simulink model "transformer_rectifier_unit"  (R2014a)
settings: Solver=FixedStepDiscrete  SolverMode=SingleTasking  StartTime=0.0  StopTime=5  FixedStep=Ts  MaxStep=1e-3  RelTol=1e-4  AbsTol=1e-4
PreLoadFcn:
  | Ts = 4e-5;
StartFcn:
  | tic;
StopFcn:
  | toc;
undefined symbols (not defined in the file or in its folder): DiscIntNeverNeededParam, param
libraries: powerlib x32, powerlib_meascontrol x5, simulink x4
settings Model: Creator=abennett  LastModifiedBy=cosorio
settings DataIOCC: SaveOutput=off  SaveTime=off  SignalLoggingName=TRU_Data
settings OptimizationCC: ExpressionDepthLimit=2147483647
settings DebuggingCC: UnderspecifiedInitializationDetection=Classic  FcnCallInpInsideContextMsg=UseLocalSettings  StateNameClashWarn=warning
settings GRTTargetCC: CombineOutputUpdateFcns=off  GRTInterface=on

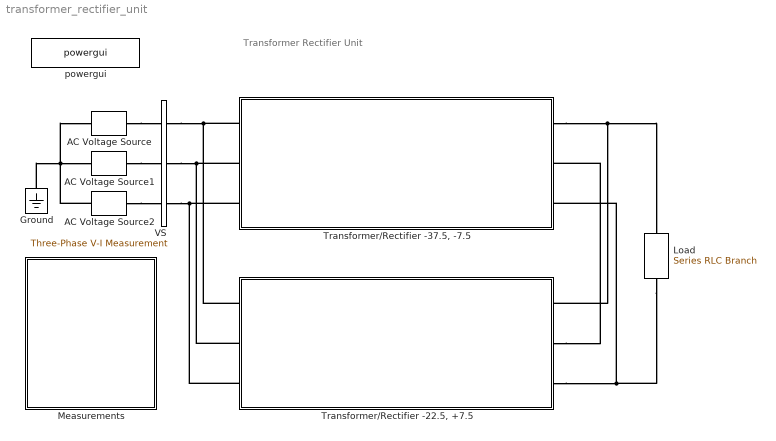
== system transformer_rectifier_unit ==
  note: Transformer Rectifier Unit
  AC Voltage Source : powerlib/Electrical Sources/AC Voltage Source  Amplitude=6600*sqrt(2)/sqrt(3)  Phase=0  Frequency=60  SampleTime=Ts  Measurements=None
  AC Voltage Source1 : powerlib/Electrical Sources/AC Voltage Source  Amplitude=6600*sqrt(2)/sqrt(3)  Phase=-120  Frequency=60  SampleTime=Ts  Measurements=None
  AC Voltage Source2 : powerlib/Electrical Sources/AC Voltage Source  Amplitude=6600*sqrt(2)/sqrt(3)  Phase=120  Frequency=60  SampleTime=Ts  Measurements=None
  Ground : powerlib/Elements/Ground  LConnTagsString=a
  Load : powerlib/Elements/Series RLC Branch  LConnTagsString=__new0  RConnTagsString=__new0  BranchType=R  Resistance=1  Inductance=1e-3  SetiL0=off  InitialCurrent=0  Capacitance=param.conv.C1  Setx0=off  InitialVoltage=0  Measurements=Branch voltage and current
  Measurements : Subsystem
  "Transformer/Rectifier -22.5, +7.5" : Subsystem
  "Transformer/Rectifier -37.5, -7.5" : Subsystem
  VS : powerlib/Measurements/Three-Phase V-I Measurement  VoltageMeasurement=phase-to-phase  SetLabelV=on  LabelV=Vsupply  Vpu=off  VpuLL=off  CurrentMeasurement=yes  SetLabelI=on  LabelI=Isupply  Ipu=off  Pbase=100e6  Vbase=500e3  OutputType=Complex  PhasorSimulation=off  PSBequivalent=0
  powergui : powerlib/powergui  Priority=1  SimulationMode=Discrete  SolverType=Tustin  SampleTime=Ts  frequency=60  SPID=off  DisableSnubberDevices=on  DisableRonSwitches=on  DisableVfSwitches=on  SwTol=0  Interpol=off  DisplayEquations=off  Ts=0  methode=off  frequencyindice=60  Pbase=100e6  ErrMax=1e-4  Iterations=50  UnitsV=kV  UnitsW=MW  FunctionMessages=off  echomessages=off  HookPort=off  EnableUseOfTLC=off  x0status=blocks  RestoreLinks=warning  ResistiveCurrentMeasurement=off  Frange=[0:2:500]  Ylog=off  Xlog=on  ShowGrid=off  save=off  variable=ZData  structure=VISupply  ZoomFFT=off  StartTime=2  cycles=10  DisplayStyle=1  fundamental=60  FreqAxis=on  MaxFrequency=3600  frequencyindicesteady=1  RmsSteady=1  display=off
  connections:
  VS/RConn1 -- "Transformer/Rectifier -22.5, +7.5"/LConn1 -- "Transformer/Rectifier -37.5, -7.5"/LConn1
  VS/RConn2 -- "Transformer/Rectifier -22.5, +7.5"/LConn2 -- "Transformer/Rectifier -37.5, -7.5"/LConn2
  VS/RConn3 -- "Transformer/Rectifier -22.5, +7.5"/LConn3 -- "Transformer/Rectifier -37.5, -7.5"/LConn3
  "Transformer/Rectifier -37.5, -7.5"/RConn1 -- Load/LConn1 -- "Transformer/Rectifier -22.5, +7.5"/RConn1
  Load/RConn1 -- "Transformer/Rectifier -22.5, +7.5"/RConn3 -- "Transformer/Rectifier -37.5, -7.5"/RConn3
  "Transformer/Rectifier -22.5, +7.5"/RConn2 -- "Transformer/Rectifier -37.5, -7.5"/RConn2
  AC Voltage Source2/RConn1 -- VS/LConn3
  AC Voltage Source1/RConn1 -- VS/LConn2
  AC Voltage Source/RConn1 -- VS/LConn1
  AC Voltage Source2/LConn1 -- Ground/LConn1 -- AC Voltage Source1/LConn1 -- AC Voltage Source/LConn1

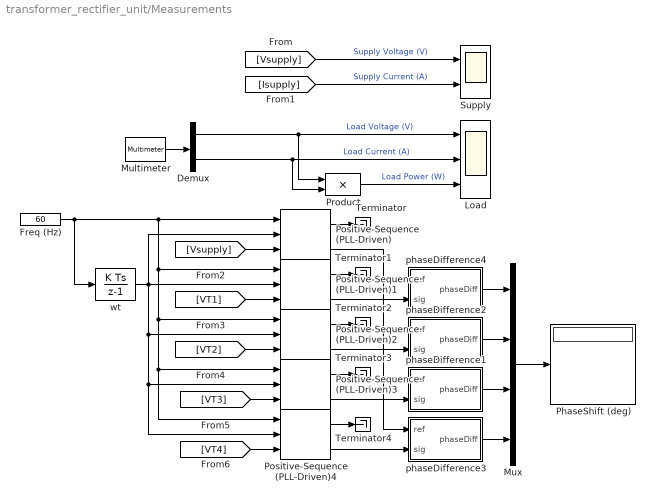
== system transformer_rectifier_unit/Measurements ==
  Demux : Demux  Outputs=2
  Freq (Hz) : Constant  Value=60
  Load : Scope  NumInputPorts=3
      settings: YMin=0~0~0  YMax=3000~3000~5000000  SaveName=VILoad
  Multimeter : powerlib/Measurements/Multimeter  PhasorSimulation=off  OutputType=Complex  sel=[1 2]  L=2  Gain=[1 1]  yselected={'Ub: Load','Ib: Load'};  PSBOutputType=1  PSBequivalent=0  AxesSetting=[0,0.1,-100,100]  Display=0  SavedBlockNames=-11
  Mux : Mux
  PhaseShift (deg) : Display
      settings: Format=bank  Decimation=100
  Positive-Sequence (PLL-Driven){,1..4} (5 alike) : powerlib_meascontrol/Measurements/Positive-Sequence (PLL-Driven)  Finit=60  Fmin=45  InInit=[1, 0]  Ts=Ts
  Product : Product  RndMeth=Zero
  Supply : Scope  NumInputPorts=2
      settings: YMin=-15000~-1000  YMax=15000~1000  SaveName=VISupply
  Terminator{,1..4} (5 alike) : Terminator
  phaseDifference1 : Subsystem
  phaseDifference2 : Subsystem
  phaseDifference3 : Subsystem
  phaseDifference4 : Subsystem
  wt : DiscreteIntegrator  gainval=2*pi  SampleTime=Ts  ICPrevOutput=DiscIntNeverNeededParam  ICPrevScaledInput=DiscIntNeverNeededParam
  wires:
  [Vsupply] -> Supply/1  "Supply Voltage (V)"
  [Isupply] -> Supply/2  "Supply Current (A)"
  Multimeter/1 -> Demux/1
  Demux/1 -> Product/1, Load/1  "Load Voltage (V)"
  Demux/2 -> Product/2, Load/2  "Load Current (A)"
  Product/1 -> Load/3  "Load Power (W)"
  [Vsupply] -> Positive-Sequence (PLL-Driven)/3
  [VT1] -> Positive-Sequence (PLL-Driven)1/3
  [VT2] -> Positive-Sequence (PLL-Driven)2/3
  [VT4] -> Positive-Sequence (PLL-Driven)4/3
  Positive-Sequence (PLL-Driven)/2 -> phaseDifference4/1(ref), phaseDifference2/1(ref), phaseDifference1/1(ref), phaseDifference3/1(ref)
  Positive-Sequence (PLL-Driven)1/2 -> phaseDifference4/2(sig)
  Positive-Sequence (PLL-Driven)2/2 -> phaseDifference2/2(sig)
  Positive-Sequence (PLL-Driven)4/2 -> phaseDifference3/2(sig)
  Positive-Sequence (PLL-Driven)/1 -> Terminator/1
  Positive-Sequence (PLL-Driven)1/1 -> Terminator1/1
  Positive-Sequence (PLL-Driven)2/1 -> Terminator2/1
  Positive-Sequence (PLL-Driven)3/1 -> Terminator3/1
  phaseDifference4/1(phaseDiff) -> Mux/1
  phaseDifference2/1(phaseDiff) -> Mux/2
  phaseDifference1/1(phaseDiff) -> Mux/3
  phaseDifference3/1(phaseDiff) -> Mux/4
  Mux/1 -> PhaseShift (deg)/1
  Positive-Sequence (PLL-Driven)4/1 -> Terminator4/1
  Positive-Sequence (PLL-Driven)3/2 -> phaseDifference1/2(sig)
  [VT3] -> Positive-Sequence (PLL-Driven)3/3
  Freq (Hz)/1 -> Positive-Sequence (PLL-Driven)4/1, Positive-Sequence (PLL-Driven)3/1, Positive-Sequence (PLL-Driven)2/1, Positive-Sequence (PLL-Driven)1/1, Positive-Sequence (PLL-Driven)/1, wt/1
  wt/1 -> Positive-Sequence (PLL-Driven)/2, Positive-Sequence (PLL-Driven)1/2, Positive-Sequence (PLL-Driven)2/2, Positive-Sequence (PLL-Driven)3/2, Positive-Sequence (PLL-Driven)4/2

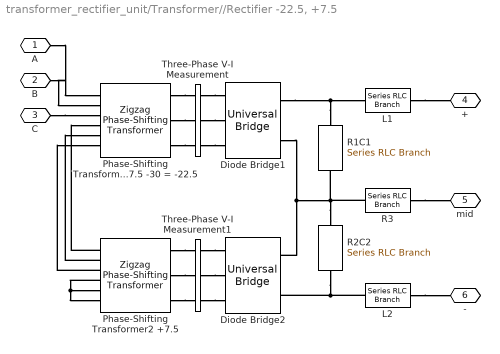
== system transformer_rectifier_unit/Transformer//Rectifier -22.5, +7.5 ==
  Diode Bridge1 : powerlib/Power Electronics/Universal Bridge  Arms=3  SnubberResistance=80  SnubberCapacitance=1e-06  Device=Diodes  Ron=1e-3  Lon=0  ForwardVoltages="[  0  0  ]"  ForwardVoltage=0  GTOparameters=[ 10e-6 , 20e-6 ]  IGBTparameters=[ 1e-6 , 2e-6 ]  Measurements=None  Measurements_2=None  converterType=Rectifier
  Diode Bridge2 : powerlib/Power Electronics/Universal Bridge  Arms=3  SnubberResistance=80  SnubberCapacitance=1e-06  Device=Diodes  Ron=1e-3  Lon=0  ForwardVoltages="[  0  0  ]"  ForwardVoltage=0  GTOparameters=[ 10e-6 , 20e-6 ]  IGBTparameters=[ 1e-6 , 2e-6 ]  Measurements=None  Measurements_2=None  converterType=Rectifier
  L1 : powerlib/Elements/Series RLC Branch  LConnTagsString=__new0  RConnTagsString=__new0  BranchType=L  Resistance=param.conv.R3  Inductance=0.005e-3  SetiL0=off  InitialCurrent=0  Capacitance=param.conv.C1  Setx0=off  InitialVoltage=0  Measurements=None
  L2 : powerlib/Elements/Series RLC Branch  LConnTagsString=__new0  RConnTagsString=__new0  BranchType=L  Resistance=param.conv.R3  Inductance=0.005e-3  SetiL0=off  InitialCurrent=0  Capacitance=param.conv.C1  Setx0=off  InitialVoltage=0  Measurements=None
  Phase-Shifting Transformer1 +7.5 -30 = -22.5 : powerlib/Elements/Zigzag Phase-Shifting Transformer  SecondaryConnection=Delta D1(-30 deg.)  UNITS=pu  NominalPower=[3300e3 60]  PrimaryVoltage=6600  SecondaryVoltage="[1725  7.5]"  Winding1=[ 0.002 0.08 ]  Winding2="[ 0.002  0.08 ]"  Winding3=[ 0.002 0.08 ]  SetSaturation=off  RmLm=[ 500 500 ]  Rm=500  Saturation=[ 0,0 ; 0.0024,1.2 ; 1.0,1.52 ]  SetInitialFlux=off  Measurements=None  InitialFluxes=[0,0,0]  MoreParameters=on  BreakLoop=off  DataType=off
  Phase-Shifting Transformer2 +7.5 : powerlib/Elements/Zigzag Phase-Shifting Transformer  SecondaryConnection=Y  UNITS=pu  NominalPower=[3300e3 60]  PrimaryVoltage=6600  SecondaryVoltage="[1725  7.5]"  Winding1=[ 0.002 0.08 ]  Winding2="[ 0.002  0.08 ]"  Winding3=[ 0.002 0.08 ]  SetSaturation=off  RmLm=[ 500 500 ]  Rm=500  Saturation=[ 0,0 ; 0.0024,1.2 ; 1.0,1.52 ]  SetInitialFlux=off  Measurements=None  InitialFluxes=[0,0,0]  MoreParameters=on  BreakLoop=off  DataType=off
  R1C1 : powerlib/Elements/Series RLC Branch  LConnTagsString=__new0  RConnTagsString=__new0  BranchType=RC  Resistance=2.5  Inductance=1e-3  SetiL0=off  InitialCurrent=0  Capacitance=10e-6  Setx0=off  InitialVoltage=0  Measurements=None
  R2C2 : powerlib/Elements/Series RLC Branch  LConnTagsString=__new0  RConnTagsString=__new0  BranchType=RC  Resistance=2.5  Inductance=1e-3  SetiL0=off  InitialCurrent=0  Capacitance=10e-6  Setx0=off  InitialVoltage=0  Measurements=None
  R3 : powerlib/Elements/Series RLC Branch  LConnTagsString=__new0  RConnTagsString=__new0  BranchType=R  Resistance=10e3  Inductance=1e-3  SetiL0=off  InitialCurrent=0  Capacitance=param.conv.C1  Setx0=off  InitialVoltage=0  Measurements=None
  Three-Phase V-I Measurement : powerlib/Measurements/Three-Phase V-I Measurement  VoltageMeasurement=phase-to-phase  SetLabelV=on  LabelV=VT3  Vpu=off  VpuLL=off  CurrentMeasurement=no  SetLabelI=off  LabelI=Iabc  Ipu=off  Pbase=100e6  Vbase=500e3  OutputType=Complex  PhasorSimulation=off  PSBequivalent=0
  Three-Phase V-I Measurement1 : powerlib/Measurements/Three-Phase V-I Measurement  VoltageMeasurement=phase-to-phase  SetLabelV=on  LabelV=VT4  Vpu=off  VpuLL=off  CurrentMeasurement=no  SetLabelI=off  LabelI=Iabc  Ipu=off  Pbase=100e6  Vbase=500e3  OutputType=Complex  PhasorSimulation=off  PSBequivalent=0
  A : PMIOPort  Port=1  Side=Left
  B : PMIOPort  Port=2  Side=Left
  C : PMIOPort  Port=3  Side=Left
  + : PMIOPort  Port=4  Side=Right
  mid : PMIOPort  Port=5  Side=Right
  - : PMIOPort  Port=6  Side=Right
  connections:
  L2/LConn1 -- -/RConn1
  L1/LConn1 -- +/RConn1
  L2/RConn1 -- R2C2/RConn1 -- Diode Bridge2/RConn2
  R1C1/LConn1 -- L1/RConn1 -- Diode Bridge1/RConn1
  R2C2/LConn1 -- R3/RConn1 -- Diode Bridge1/RConn2 -- Diode Bridge2/RConn1 -- R1C1/RConn1
  R3/LConn1 -- mid/RConn1
  Phase-Shifting Transformer2 +7.5/LConn4 -- Phase-Shifting Transformer2 +7.5/LConn6 -- Phase-Shifting Transformer2 +7.5/LConn5
  C/RConn1 -- Phase-Shifting Transformer1 +7.5 -30 = -22.5/LConn3
  B/RConn1 -- Phase-Shifting Transformer1 +7.5 -30 = -22.5/LConn2
  Phase-Shifting Transformer2 +7.5/LConn2 -- Phase-Shifting Transformer1 +7.5 -30 = -22.5/LConn5
  Phase-Shifting Transformer2 +7.5/LConn3 -- Phase-Shifting Transformer1 +7.5 -30 = -22.5/LConn6
  Phase-Shifting Transformer2 +7.5/LConn1 -- Phase-Shifting Transformer1 +7.5 -30 = -22.5/LConn4
  A/RConn1 -- Phase-Shifting Transformer1 +7.5 -30 = -22.5/LConn1
  Phase-Shifting Transformer1 +7.5 -30 = -22.5/RConn1 -- Three-Phase V-I Measurement/LConn1
  Phase-Shifting Transformer1 +7.5 -30 = -22.5/RConn2 -- Three-Phase V-I Measurement/LConn2
  Phase-Shifting Transformer1 +7.5 -30 = -22.5/RConn3 -- Three-Phase V-I Measurement/LConn3
  Three-Phase V-I Measurement/RConn1 -- Diode Bridge1/LConn1
  Three-Phase V-I Measurement/RConn2 -- Diode Bridge1/LConn2
  Three-Phase V-I Measurement/RConn3 -- Diode Bridge1/LConn3
  Phase-Shifting Transformer2 +7.5/RConn2 -- Three-Phase V-I Measurement1/LConn2
  Phase-Shifting Transformer2 +7.5/RConn3 -- Three-Phase V-I Measurement1/LConn3
  Phase-Shifting Transformer2 +7.5/RConn1 -- Three-Phase V-I Measurement1/LConn1
  Three-Phase V-I Measurement1/RConn3 -- Diode Bridge2/LConn3
  Three-Phase V-I Measurement1/RConn2 -- Diode Bridge2/LConn2
  Three-Phase V-I Measurement1/RConn1 -- Diode Bridge2/LConn1

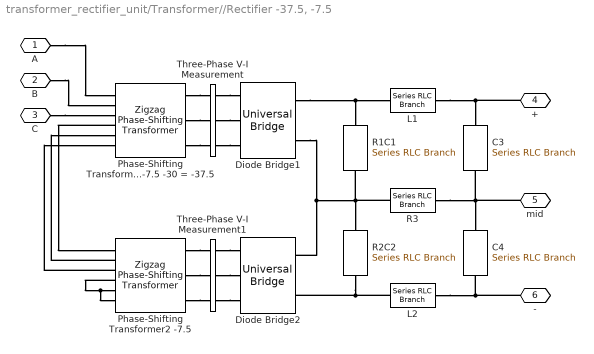
== system transformer_rectifier_unit/Transformer//Rectifier -37.5, -7.5 ==
  C3 : powerlib/Elements/Series RLC Branch  LConnTagsString=__new0  RConnTagsString=__new0  BranchType=C  Resistance=param.conv.R1  Inductance=1e-3  SetiL0=off  InitialCurrent=0  Capacitance=9.6e-3  Setx0=off  InitialVoltage=0  Measurements=None
  C4 : powerlib/Elements/Series RLC Branch  LConnTagsString=__new0  RConnTagsString=__new0  BranchType=C  Resistance=param.conv.R1  Inductance=1e-3  SetiL0=off  InitialCurrent=0  Capacitance=9.6e-3  Setx0=off  InitialVoltage=0  Measurements=None
  Diode Bridge1 : powerlib/Power Electronics/Universal Bridge  Arms=3  SnubberResistance=80  SnubberCapacitance=1e-06  Device=Diodes  Ron=1e-3  Lon=0  ForwardVoltages="[  0  0  ]"  ForwardVoltage=0  GTOparameters=[ 10e-6 , 20e-6 ]  IGBTparameters=[ 1e-6 , 2e-6 ]  Measurements=None  Measurements_2=None  converterType=Rectifier
  Diode Bridge2 : powerlib/Power Electronics/Universal Bridge  Arms=3  SnubberResistance=80  SnubberCapacitance=1e-06  Device=Diodes  Ron=1e-3  Lon=0  ForwardVoltages="[  0  0  ]"  ForwardVoltage=0  GTOparameters=[ 10e-6 , 20e-6 ]  IGBTparameters=[ 1e-6 , 2e-6 ]  Measurements=None  Measurements_2=None  converterType=Rectifier
  L1 : powerlib/Elements/Series RLC Branch  LConnTagsString=__new0  RConnTagsString=__new0  BranchType=L  Resistance=param.conv.R3  Inductance=0.005e-3  SetiL0=off  InitialCurrent=0  Capacitance=param.conv.C1  Setx0=off  InitialVoltage=0  Measurements=None
  L2 : powerlib/Elements/Series RLC Branch  LConnTagsString=__new0  RConnTagsString=__new0  BranchType=L  Resistance=param.conv.R3  Inductance=0.005e-3  SetiL0=off  InitialCurrent=0  Capacitance=param.conv.C1  Setx0=off  InitialVoltage=0  Measurements=None
  Phase-Shifting Transformer1 -7.5 -30 = -37.5 : powerlib/Elements/Zigzag Phase-Shifting Transformer  SecondaryConnection=Delta D1(-30 deg.)  UNITS=pu  NominalPower=[3300e3 60]  PrimaryVoltage=6600  SecondaryVoltage="[1725  -7.5]"  Winding1=[ 0.002 0.08 ]  Winding2="[ 0.002  0.08 ]"  Winding3=[ 0.002 0.08 ]  SetSaturation=off  RmLm=[ 500 500 ]  Rm=500  Saturation=[ 0,0 ; 0.0024,1.2 ; 1.0,1.52 ]  SetInitialFlux=off  Measurements=None  InitialFluxes=[0,0,0]  MoreParameters=on  BreakLoop=off  DataType=off
  Phase-Shifting Transformer2 -7.5 : powerlib/Elements/Zigzag Phase-Shifting Transformer  SecondaryConnection=Y  UNITS=pu  NominalPower=[3300e3 60]  PrimaryVoltage=6600  SecondaryVoltage="[1725  -7.5]"  Winding1=[ 0.002 0.08 ]  Winding2="[ 0.002  0.08 ]"  Winding3=[ 0.002 0.08 ]  SetSaturation=off  RmLm=[ 500 500 ]  Rm=500  Saturation=[ 0,0 ; 0.0024,1.2 ; 1.0,1.52 ]  SetInitialFlux=off  Measurements=None  InitialFluxes=[0,0,0]  MoreParameters=on  BreakLoop=off  DataType=off
  R1C1 : powerlib/Elements/Series RLC Branch  LConnTagsString=__new0  RConnTagsString=__new0  BranchType=RC  Resistance=2.5  Inductance=1e-3  SetiL0=off  InitialCurrent=0  Capacitance=10e-6  Setx0=off  InitialVoltage=0  Measurements=None
  R2C2 : powerlib/Elements/Series RLC Branch  LConnTagsString=__new0  RConnTagsString=__new0  BranchType=RC  Resistance=2.5  Inductance=1e-3  SetiL0=off  InitialCurrent=0  Capacitance=10e-6  Setx0=off  InitialVoltage=0  Measurements=None
  R3 : powerlib/Elements/Series RLC Branch  LConnTagsString=__new0  RConnTagsString=__new0  BranchType=R  Resistance=10e3  Inductance=1e-3  SetiL0=off  InitialCurrent=0  Capacitance=param.conv.C1  Setx0=off  InitialVoltage=0  Measurements=None
  Three-Phase V-I Measurement : powerlib/Measurements/Three-Phase V-I Measurement  VoltageMeasurement=phase-to-phase  SetLabelV=on  LabelV=VT1  Vpu=off  VpuLL=off  CurrentMeasurement=no  SetLabelI=off  LabelI=Iabc  Ipu=off  Pbase=100e6  Vbase=500e3  OutputType=Complex  PhasorSimulation=off  PSBequivalent=0
  Three-Phase V-I Measurement1 : powerlib/Measurements/Three-Phase V-I Measurement  VoltageMeasurement=phase-to-phase  SetLabelV=on  LabelV=VT2  Vpu=off  VpuLL=off  CurrentMeasurement=no  SetLabelI=off  LabelI=Iabc  Ipu=off  Pbase=100e6  Vbase=500e3  OutputType=Complex  PhasorSimulation=off  PSBequivalent=0
  A : PMIOPort  Port=1  Side=Left
  B : PMIOPort  Port=2  Side=Left
  C : PMIOPort  Port=3  Side=Left
  + : PMIOPort  Port=4  Side=Right
  mid : PMIOPort  Port=5  Side=Right
  - : PMIOPort  Port=6  Side=Right
  connections:
  Diode Bridge1/RConn2 -- R3/RConn1 -- R2C2/LConn1 -- R1C1/RConn1 -- Diode Bridge2/RConn1
  Diode Bridge1/RConn1 -- L1/RConn1 -- R1C1/LConn1
  R2C2/RConn1 -- L2/RConn1 -- Diode Bridge2/RConn2
  L1/LConn1 -- +/RConn1 -- C3/LConn1
  R3/LConn1 -- mid/RConn1 -- C3/RConn1 -- C4/LConn1
  L2/LConn1 -- -/RConn1 -- C4/RConn1
  Phase-Shifting Transformer2 -7.5/LConn5 -- Phase-Shifting Transformer2 -7.5/LConn6 -- Phase-Shifting Transformer2 -7.5/LConn4
  A/RConn1 -- Phase-Shifting Transformer1 -7.5 -30 = -37.5/LConn1
  B/RConn1 -- Phase-Shifting Transformer1 -7.5 -30 = -37.5/LConn2
  C/RConn1 -- Phase-Shifting Transformer1 -7.5 -30 = -37.5/LConn3
  Phase-Shifting Transformer1 -7.5 -30 = -37.5/LConn4 -- Phase-Shifting Transformer2 -7.5/LConn1
  Phase-Shifting Transformer2 -7.5/LConn2 -- Phase-Shifting Transformer1 -7.5 -30 = -37.5/LConn5
  Phase-Shifting Transformer2 -7.5/LConn3 -- Phase-Shifting Transformer1 -7.5 -30 = -37.5/LConn6
  Phase-Shifting Transformer1 -7.5 -30 = -37.5/RConn3 -- Three-Phase V-I Measurement/LConn3
  Phase-Shifting Transformer1 -7.5 -30 = -37.5/RConn2 -- Three-Phase V-I Measurement/LConn2
  Phase-Shifting Transformer1 -7.5 -30 = -37.5/RConn1 -- Three-Phase V-I Measurement/LConn1
  Three-Phase V-I Measurement/RConn1 -- Diode Bridge1/LConn1
  Three-Phase V-I Measurement/RConn2 -- Diode Bridge1/LConn2
  Three-Phase V-I Measurement/RConn3 -- Diode Bridge1/LConn3
  Phase-Shifting Transformer2 -7.5/RConn3 -- Three-Phase V-I Measurement1/LConn3
  Phase-Shifting Transformer2 -7.5/RConn1 -- Three-Phase V-I Measurement1/LConn1
  Phase-Shifting Transformer2 -7.5/RConn2 -- Three-Phase V-I Measurement1/LConn2
  Three-Phase V-I Measurement1/RConn1 -- Diode Bridge2/LConn1
  Three-Phase V-I Measurement1/RConn2 -- Diode Bridge2/LConn2
  Three-Phase V-I Measurement1/RConn3 -- Diode Bridge2/LConn3

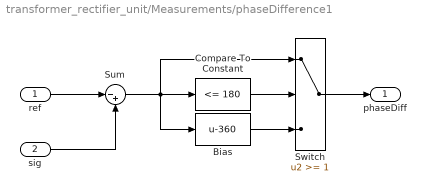
== system transformer_rectifier_unit/Measurements/phaseDifference1 ==
  ref : Inport
  sig : Inport  Port=2
  Bias : Bias  Bias=-360
  Compare To Constant : simulink/Logic and Bit Operations/Compare To Constant  relop=<=  const=180  OutDataTypeStr=boolean
  Sum : Sum  Inputs=|-+  SaturateOnIntegerOverflow=on  InputSameDT=on  OutDataTypeStr=Inherit: Same as first input
  Switch : Switch  Threshold=1
  phaseDiff : Outport
  wires:
  Sum/1 -> Bias/1, Compare To Constant/1, Switch/1
  sig/1 -> Sum/2
  ref/1 -> Sum/1
  Switch/1 -> phaseDiff/1
  Bias/1 -> Switch/3
  Compare To Constant/1 -> Switch/2

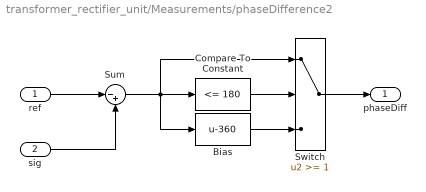
== system transformer_rectifier_unit/Measurements/phaseDifference2 ==
  ref : Inport
  sig : Inport  Port=2
  Bias : Bias  Bias=-360
  Compare To Constant : simulink/Logic and Bit Operations/Compare To Constant  relop=<=  const=180  OutDataTypeStr=boolean
  Sum : Sum  Inputs=|-+  SaturateOnIntegerOverflow=on  InputSameDT=on  OutDataTypeStr=Inherit: Same as first input
  Switch : Switch  Threshold=1
  phaseDiff : Outport
  wires:
  Compare To Constant/1 -> Switch/2
  Bias/1 -> Switch/3
  Switch/1 -> phaseDiff/1
  ref/1 -> Sum/1
  sig/1 -> Sum/2
  Sum/1 -> Switch/1, Compare To Constant/1, Bias/1

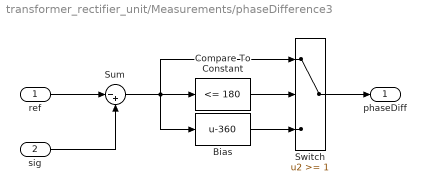
== system transformer_rectifier_unit/Measurements/phaseDifference3 ==
  ref : Inport
  sig : Inport  Port=2
  Bias : Bias  Bias=-360
  Compare To Constant : simulink/Logic and Bit Operations/Compare To Constant  relop=<=  const=180  OutDataTypeStr=boolean
  Sum : Sum  Inputs=|-+  SaturateOnIntegerOverflow=on  InputSameDT=on  OutDataTypeStr=Inherit: Same as first input
  Switch : Switch  Threshold=1
  phaseDiff : Outport
  wires:
  Compare To Constant/1 -> Switch/2
  Bias/1 -> Switch/3
  Switch/1 -> phaseDiff/1
  ref/1 -> Sum/1
  sig/1 -> Sum/2
  Sum/1 -> Switch/1, Compare To Constant/1, Bias/1

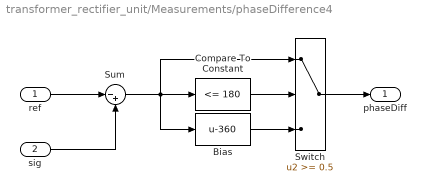
== system transformer_rectifier_unit/Measurements/phaseDifference4 ==
  ref : Inport
  sig : Inport  Port=2
  Bias : Bias  Bias=-360
  Compare To Constant : simulink/Logic and Bit Operations/Compare To Constant  relop=<=  const=180  OutDataTypeStr=boolean
  Sum : Sum  Inputs=|-+  SaturateOnIntegerOverflow=on  InputSameDT=on  OutDataTypeStr=Inherit: Same as first input
  Switch : Switch  Threshold=0.5  SampleTime=Ts
  phaseDiff : Outport
  wires:
  Sum/1 -> Bias/1, Compare To Constant/1, Switch/1
  sig/1 -> Sum/2
  ref/1 -> Sum/1
  Switch/1 -> phaseDiff/1
  Bias/1 -> Switch/3
  Compare To Constant/1 -> Switch/2
